simulink model "DSF_Activation_Requester"  (R2017b)
settings: configuration reference "CommonModelConfiguration" (kept outside this file)
undefined symbols (not defined in the file): cc_param_23, cc_param_36, LCFG_ActivationDeactivation
settings Model: Creator=RPETE142  LastModifiedBy=RKALLUM
settings ConfigSetRef: SourceLocation=Base Workspace

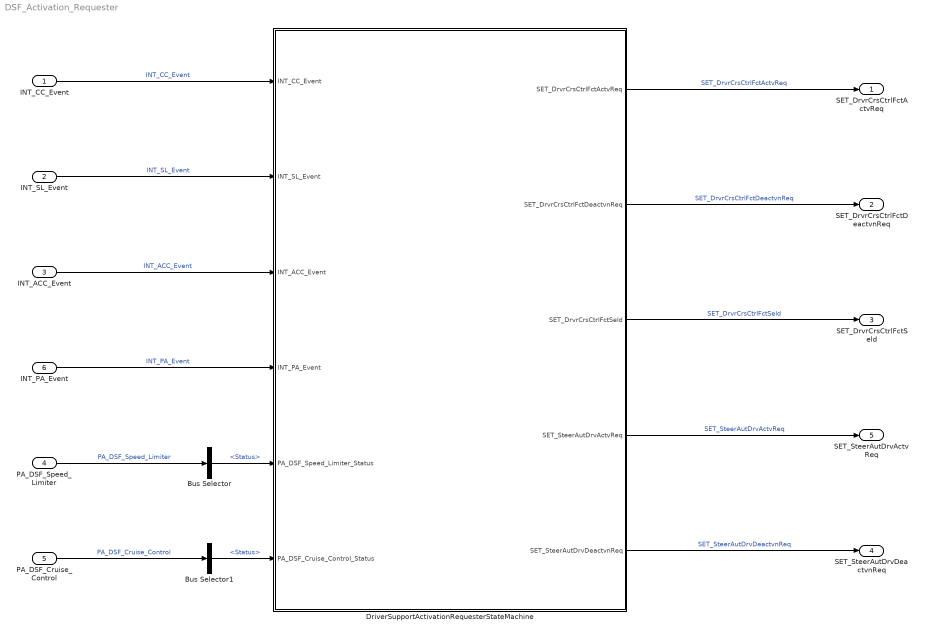
== system DSF_Activation_Requester ==
  INT_CC_Event : Inport  OutDataTypeStr=Enum: E_DSF_Event
  INT_SL_Event : Inport  Port=2  OutDataTypeStr=Enum: E_DSF_Event
  INT_ACC_Event : Inport  Port=3  OutDataTypeStr=Enum: E_DSF_Event
  PA_DSF_Speed_Limiter : Inport  Port=4  OutDataTypeStr=Bus: PA_DSF
  PA_DSF_Cruise_Control : Inport  Port=5  OutDataTypeStr=Bus: PA_DSF
  INT_PA_Event : Inport  Port=6  OutDataTypeStr=Enum: E_DSF_Event
  Bus Selector : BusSelector  OutputSignals=Status
  Bus Selector1 : BusSelector  OutputSignals=Status
  "DriverSupportActivationRequesterStateMachine " : Stateflow chart  TreatAsAtomicUnit=on
  SET_DrvrCrsCtrlFctActvReq : Outport  OutDataTypeStr=Enum: OnOff1
  SET_DrvrCrsCtrlFctDeactvnReq : Outport  Port=2  OutDataTypeStr=Enum: OnOff1
  SET_DrvrCrsCtrlFctSeld : Outport  Port=3  OutDataTypeStr=Enum: DrvrCrsCtrlFctSeldTyp
  SET_SteerAutDrvDeactvnReq : Outport  Port=4  OutDataTypeStr=Enum: NoYesCrit1
  SET_SteerAutDrvActvReq : Outport  Port=5  OutDataTypeStr=Enum: NoYesCrit1
  wires:
  INT_CC_Event/1 -> "DriverSupportActivationRequesterStateMachine "/1(INT_CC_Event)  "INT_CC_Event"
  INT_SL_Event/1 -> "DriverSupportActivationRequesterStateMachine "/2(INT_SL_Event)  "INT_SL_Event"
  INT_ACC_Event/1 -> "DriverSupportActivationRequesterStateMachine "/3(INT_ACC_Event)  "INT_ACC_Event"
  PA_DSF_Speed_Limiter/1 -> Bus Selector/1  "PA_DSF_Speed_Limiter"
  PA_DSF_Cruise_Control/1 -> Bus Selector1/1  "PA_DSF_Cruise_Control"
  "DriverSupportActivationRequesterStateMachine "/1(SET_DrvrCrsCtrlFctActvReq) -> SET_DrvrCrsCtrlFctActvReq/1  "SET_DrvrCrsCtrlFctActvReq"
  "DriverSupportActivationRequesterStateMachine "/2(SET_DrvrCrsCtrlFctDeactvnReq) -> SET_DrvrCrsCtrlFctDeactvnReq/1  "SET_DrvrCrsCtrlFctDeactvnReq"
  "DriverSupportActivationRequesterStateMachine "/3(SET_DrvrCrsCtrlFctSeld) -> SET_DrvrCrsCtrlFctSeld/1  "SET_DrvrCrsCtrlFctSeld"
  Bus Selector/1 -> "DriverSupportActivationRequesterStateMachine "/5(PA_DSF_Speed_Limiter_Status)  "<Status>"
  Bus Selector1/1 -> "DriverSupportActivationRequesterStateMachine "/6(PA_DSF_Cruise_Control_Status)  "<Status>"
  "DriverSupportActivationRequesterStateMachine "/5(SET_SteerAutDrvDeactvnReq) -> SET_SteerAutDrvDeactvnReq/1  "SET_SteerAutDrvDeactvnReq"
  "DriverSupportActivationRequesterStateMachine "/4(SET_SteerAutDrvActvReq) -> SET_SteerAutDrvActvReq/1  "SET_SteerAutDrvActvReq"
  INT_PA_Event/1 -> "DriverSupportActivationRequesterStateMachine "/4(INT_PA_Event)  "INT_PA_Event"

== stateflow chart DSF_Activation_Requester/DriverSupportActivationRequesterStateMachine  ==
  state CARCONFIG_INVALID
    entry:
    SET_DrvrCrsCtrlFctSeld = DrvrCrsCtrlFctSeldTyp.DrvrCrsCtrlFctSeldTyp_Off;
    SET_DrvrCrsCtrlFctActvReq = OnOff1.OnOff1_Off;
    SET_DrvrCrsCtrlFctDeactvnReq = OnOff1.OnOff1_Off;
  state SYSTEM_OK
    state CRUISE_FUNCTIONS [parallel]
      entry: SET_DrvrCrsCtrlFctSeld = DrvrCrsCtrlFctSeldTyp.DrvrCrsCtrlFctSeldTyp_Off;
      settings: executionOrder=1
      state ACTIVATION
        entry: SET_DrvrCrsCtrlFctActvReq = OnOff1.OnOff1_On;
        SET_DrvrCrsCtrlFctDeactvnReq = OnOff1.OnOff1_Off;
      state NO_REQUESTS
        entry:
        SET_DrvrCrsCtrlFctActvReq = OnOff1.OnOff1_Off;
        SET_DrvrCrsCtrlFctDeactvnReq = OnOff1.OnOff1_Off;
      state DEACTIVATION
        entry: SET_DrvrCrsCtrlFctDeactvnReq = OnOff1.OnOff1_On;
        SET_DrvrCrsCtrlFctActvReq = OnOff1.OnOff1_Off;
      state cDeactivation = cruiseDeactivation [function]
        (default) -> (junction 1551)
        (junction 1551) -> (junction 1559) [order 1] : [hasChangedTo(INT_CC_Event,E_DSF_Event.Deactivation) ||...
            | hasChangedTo(INT_SL_Event,E_DSF_Event.Deactivation) ||...
            | hasChangedTo(INT_ACC_Event,E_DSF_Event.Deactivation)]
        (junction 1559) -> (junction 1658) : {cDeactivation = true;}
        (junction 1551) -> (junction 1566) [order 2] : {cDeactivation = false;}
        (junction 1658) -> (junction 1566)
        (junction 1566) -> (junction 1570)
      state cActivation = cruiseActivation [function]
        (default) -> (junction 1494)
        (junction 1494) -> (junction 1507) [order 1] : [PA_DSF_Cruise_Control_Status == E_CommonStatus.Available]
            | {SET_DrvrCrsCtrlFctSeld = DrvrCrsCtrlFctSeldTyp.DrvrCrsCtrlFctSeldTyp_CrsCtrlFct;}
        (junction 1494) -> (junction 1506) [order 2] : [PA_DSF_Speed_Limiter_Status == E_CommonStatus.Available]
            | {SET_DrvrCrsCtrlFctSeld = DrvrCrsCtrlFctSeldTyp.DrvrCrsCtrlFctSeldTyp_SpdLimFct;}
        (junction 1507) -> (junction 1515) [order 2]
        (junction 1506) -> (junction 1521) [order 2]
        (junction 1507) -> (junction 1537) [order 1] : [hasChangedTo(INT_CC_Event,E_DSF_Event.Activation) ||...
            | hasChangedTo(INT_CC_Event,E_DSF_Event.Resume)]
            | {cActivation = true;
            | }
        (junction 1506) -> (junction 1533) [order 1] : [hasChangedTo(INT_SL_Event,E_DSF_Event.Activation) ||...
            | hasChangedTo(INT_SL_Event,E_DSF_Event.Resume)]
            | {cActivation = true;
            | }
        (junction 1515) -> (junction 1539) : {cActivation = false;}
        (junction 1521) -> (junction 1535) : {cActivation = false;}
        (junction 1494) -> (junction 1504) [order 3] : {SET_DrvrCrsCtrlFctSeld = DrvrCrsCtrlFctSeldTyp.DrvrCrsCtrlFctSeldTyp_AccFct;}
        (junction 1504) -> (junction 1525) [order 1] : [hasChangedTo(INT_ACC_Event,E_DSF_Event.Activation) ||...
            | hasChangedTo(INT_ACC_Event,E_DSF_Event.Resume)]
            | {cActivation = true;
            | }
        (junction 1504) -> (junction 1527) [order 2] : {cActivation = false;}
        (junction 1525) -> (junction 1529)
        (junction 1527) -> (junction 1531)
        (junction 1535) -> (junction 1533)
        (junction 1533) -> (junction 1531)
        (junction 1539) -> (junction 1537)
        (junction 1537) -> (junction 1529)
        (junction 1529) -> (junction 1544)
        (junction 1531) -> (junction 1544)
        (junction 1544) -> (junction 1548)
      (default) -> SYSTEM_OK.CRUISE_FUNCTIONS.NO_REQUESTS
      SYSTEM_OK.CRUISE_FUNCTIONS.NO_REQUESTS -> SYSTEM_OK.CRUISE_FUNCTIONS.ACTIVATION [order 1] : [cruiseActivation()]
      SYSTEM_OK.CRUISE_FUNCTIONS.ACTIVATION -> SYSTEM_OK.CRUISE_FUNCTIONS.NO_REQUESTS [order 1] : [after(LCFG_ActivationDeactivation,sec)]
      SYSTEM_OK.CRUISE_FUNCTIONS.DEACTIVATION -> SYSTEM_OK.CRUISE_FUNCTIONS.ACTIVATION [order 2] : [cruiseActivation()]
      SYSTEM_OK.CRUISE_FUNCTIONS.ACTIVATION -> SYSTEM_OK.CRUISE_FUNCTIONS.DEACTIVATION [order 2] : [cruiseDeactivation()]
      SYSTEM_OK.CRUISE_FUNCTIONS.NO_REQUESTS -> SYSTEM_OK.CRUISE_FUNCTIONS.DEACTIVATION [order 2] : [cruiseDeactivation()]
      SYSTEM_OK.CRUISE_FUNCTIONS.DEACTIVATION -> SYSTEM_OK.CRUISE_FUNCTIONS.NO_REQUESTS [order 1] : [after(LCFG_ActivationDeactivation,sec)]
    state PILOT_ASSIST [parallel]
      settings: executionOrder=2
      state ACTIVATION
        entry:
        SET_SteerAutDrvActvReq = NoYesCrit1.NoYesCrit1_Yes;
        SET_SteerAutDrvDeactvnReq = NoYesCrit1.NoYesCrit1_No;
      state NO_REQUESTS
        entry:
        SET_SteerAutDrvActvReq = NoYesCrit1.NoYesCrit1_No;
        SET_SteerAutDrvDeactvnReq = NoYesCrit1.NoYesCrit1_No;
      state DEACTIVATION
        entry:
        SET_SteerAutDrvActvReq = NoYesCrit1.NoYesCrit1_No;
        SET_SteerAutDrvDeactvnReq = NoYesCrit1.NoYesCrit1_Yes;
      (default) -> SYSTEM_OK.PILOT_ASSIST.NO_REQUESTS
      SYSTEM_OK.PILOT_ASSIST.NO_REQUESTS -> SYSTEM_OK.PILOT_ASSIST.ACTIVATION [order 1] : [hasChangedTo(INT_PA_Event,E_DSF_Event.Activation)]
      SYSTEM_OK.PILOT_ASSIST.ACTIVATION -> SYSTEM_OK.PILOT_ASSIST.NO_REQUESTS [order 1] : [after(LCFG_ActivationDeactivation,sec)]
      SYSTEM_OK.PILOT_ASSIST.DEACTIVATION -> SYSTEM_OK.PILOT_ASSIST.ACTIVATION [order 2] : [hasChangedTo(INT_PA_Event,E_DSF_Event.Activation)]
      SYSTEM_OK.PILOT_ASSIST.ACTIVATION -> SYSTEM_OK.PILOT_ASSIST.DEACTIVATION [order 2] : [hasChangedTo(INT_PA_Event,E_DSF_Event.Deactivation)]
      SYSTEM_OK.PILOT_ASSIST.NO_REQUESTS -> SYSTEM_OK.PILOT_ASSIST.DEACTIVATION [order 2] : [hasChangedTo(INT_PA_Event,E_DSF_Event.Deactivation)]
      SYSTEM_OK.PILOT_ASSIST.DEACTIVATION -> SYSTEM_OK.PILOT_ASSIST.NO_REQUESTS [order 1] : [after(LCFG_ActivationDeactivation,sec)]
  (default) -> (junction 284)
  (junction 284) -> CARCONFIG_INVALID [order 2]
  (junction 284) -> SYSTEM_OK [order 1] : [cc_param_23 > 1 || cc_param_36>1]
  data: cDeactivation function_output; cActivation function_output; SET_DrvrCrsCtrlFctActvReq output Enum: OnOff1; INT_CC_Event input Enum: E_DSF_Event; INT_SL_Event input Enum: E_DSF_Event; INT_ACC_Event input Enum: E_DSF_Event; INT_PA_Event input Enum: E_DSF_Event; SET_DrvrCrsCtrlFctDeactvnReq output Enum: OnOff1; cc_param_36 parameter; cc_param_23 parameter; PA_DSF_Speed_Limiter_Status input Enum: E_CommonStatus; PA_DSF_Cruise_Control_Status input Enum: E_CommonStatus; LCFG_ActivationDeactivation parameter; SET_DrvrCrsCtrlFctSeld output Enum: DrvrCrsCtrlFctSeldTyp; SET_SteerAutDrvActvReq output Enum: NoYesCrit1; SET_SteerAutDrvDeactvnReq output Enum: NoYesCrit1
